simulink model "ktrgk"  (R2017b)
settings: Solver=FixedStepAuto  StartTime=0.0  StopTime=10.0  RelTol=1e-3
settings Model: Creator=DELL  LastModifiedBy=DELL

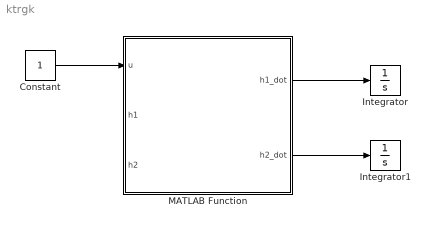
== system ktrgk ==
  Constant : Constant
  Integrator : Integrator  InitialCondition=0.01
  Integrator1 : Integrator  InitialCondition=0.01
  MATLAB Function : MATLAB Function  TreatAsAtomicUnit=on
  wires:
  MATLAB Function/1(h1_dot) -> Integrator/1
  MATLAB Function/2(h2_dot) -> Integrator1/1
  Constant/1 -> MATLAB Function/1(u)

== matlab function ktrgk/MATLAB Function ==
  data: u input; h1_dot output; h1 input; h2 input; h2_dot output
function [h1_dot, h2_dot] = fcn(u,h1,h2)

%#codegen
A1 = 175;      % cm^2
A2 = 154;      % cm^2
b1 = 1.1;      % cm^2
b2 = 1.0;      % cm^2
K = 41;        % cm^3/s/V
C = 0.6;
g = 981;       % cm/s^2
h1_dot=(K*u-sign(h1-h2)*b1*C*sqrt(2*g*abs(h1-h2)))/A1;
h2_dot=(sign(h1-h2)*b1*C*sqrt(2*g*abs(h1-h2))-b2*C*sqrt(2*g*h2))/A2;
